simulink model "Test_Model"  (R2023b)
settings: Solver=FixedStepDiscrete  StartTime=0.0  StopTime=30  FixedStep=0.01  RelTol=1e-3
settings Model: Creator=MrLove  LastModifiedBy=MrLove

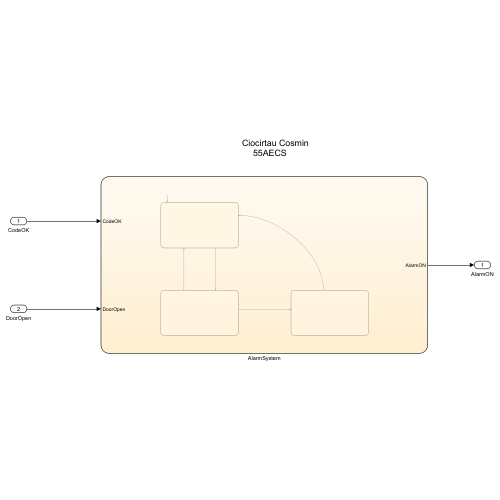
[thumbnail: Simulink's stored preview of the top-level diagram]
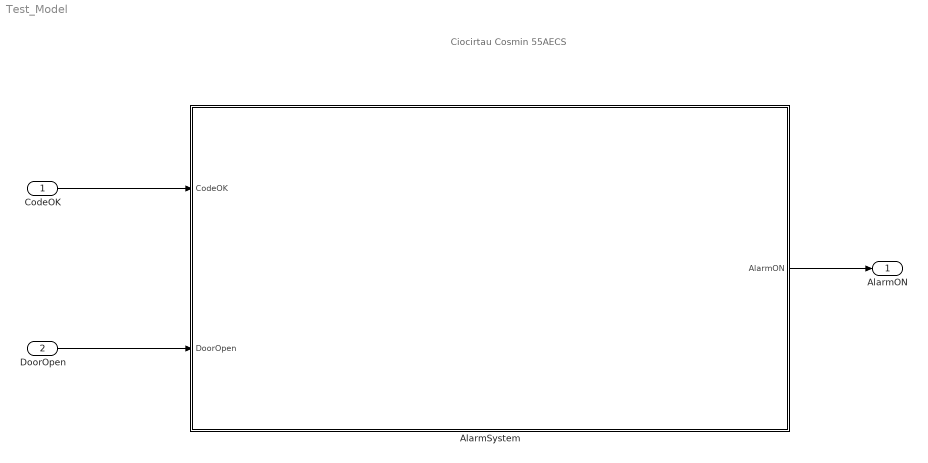
== system Test_Model ==
  note: Ciocirtau Cosmin
      | 55AECS
  CodeOK : Inport
  DoorOpen : Inport  Port=2
  AlarmSystem : Stateflow chart  TreatAsAtomicUnit=on
  AlarmON : Outport
  wires:
  AlarmSystem/1(AlarmON) -> AlarmON/1
  CodeOK/1 -> AlarmSystem/1(CodeOK)
  DoorOpen/1 -> AlarmSystem/2(DoorOpen)

== stateflow chart Test_Model/AlarmSystem ==
  state IDLE
    en:
    AlarmON = false;
  state WAIT
  state ALARM
    en:
    AlarmON = true;
  (default) -> IDLE
  ALARM -> IDLE : [CodeOK == true]
  WAIT -> IDLE [order 1] : [CodeOK == true]
  IDLE -> WAIT : [DoorOpen == true]
  WAIT -> ALARM [order 2] : [after(15,sec)]
  data: CodeOK input; DoorOpen input; AlarmON output
